simulink model "singletrack_ideal_model_ROS"  (R2018b)
settings: Solver=VariableStepAuto  StartTime=0.0  StopTime=20.0  FixedStep=1e-5  RelTol=1e-3
model workspace (MAT data in the model file):
  SL_ROS_VariableLengthArrays_MaxSizes.CommonInfo.ArrayTruncateAction = 'EmitWarning'
  SL_ROS_VariableLengthArrays_MaxSizes.MsgTypeMap = containers.Map
  SL_ROS_VariableLengthArrays_MaxSizes.MsgTypeMap.serialization.keys = {}
  SL_ROS_VariableLengthArrays_MaxSizes.MsgTypeMap.serialization.values = {}
  SL_ROS_VariableLengthArrays_MaxSizes.MsgTypeMap.serialization.uniformity = 0
  SL_ROS_VariableLengthArrays_MaxSizes.MsgTypeMap.serialization.keyType = 'char'
  SL_ROS_VariableLengthArrays_MaxSizes.MsgTypeMap.serialization.valueType = 'any'
values from neighbouring files (symbols this model uses):
  car_param = [a, b, Cf, Cr, Iz, m]    [init_singletrack.m]
  car_state0 = [psi0, r0, beta0, x0, y0]    [init_singletrack.m]
  fblin_Ts = 0.01    [init_singletrack.m]
  meas_Ts = 0.001    [init_singletrack.m]
  P = 0.5    [init_singletrack.m]    (also in init_unicycle.m)
  ROS_clockPublishingPeriod = 1.0e-2    (= 0.01)    [initParameters.m]    (also in init_singletrack.m = 0.0005)
  ROS_statePublishingPeriod = 2.0e-2    (= 0.02)    [initParameters.m]    (also in init_singletrack.m = 0.01)
undefined symbols (not defined in the file or in its folder): Clock_, fblin_output_singletrack_lopez1, fblin_output_singletrack_lopez2, fblin_output_singletrack_spaliviero, fblin_outputInverse_singletrack_lopez1, fblin_outputInverse_singletrack_lopez2, fblin_outputInverse_singletrack_spaliviero, Sideslip, singleTrack_model, Theta, Vx, Vy, X, Y
libraries: robotlib x14
settings Model: Creator=bascetta  LastModifiedBy=bascetta
settings SFSimCC: SimUseLocalCustomCode=off
settings RTWCC: RTWUseLocalCustomCode=off

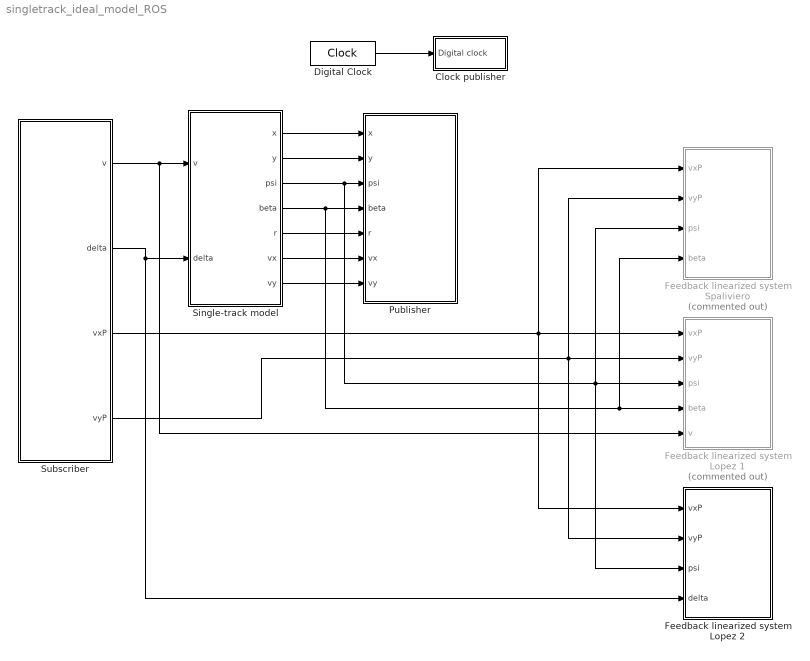
== system singletrack_ideal_model_ROS ==
  Clock publisher : Subsystem
  Digital Clock : DigitalClock  SampleTime=ROS_clockPublishingPeriod
  Feedback linearized system Lopez 1 : Subsystem  Commented=on
  Feedback linearized system Lopez 2 : Subsystem
  Feedback linearized system Spaliviero : Subsystem  Commented=on
  Publisher : Subsystem
  Single-track model : Subsystem  mask{car_parameters=car_param, car_state0=car_state0}
      mask prompts: car_parameters "Car parameters"; car_state0 "Car initial state"
  Subscriber : Subsystem
  wires:
  Single-track model/3(psi) -> Feedback linearized system Lopez 2/3(psi), Feedback linearized system Spaliviero/3(psi), Feedback linearized system Lopez 1/3(psi), Publisher/3(psi)
  Single-track model/4(beta) -> Feedback linearized system Spaliviero/4(beta), Feedback linearized system Lopez 1/4(beta), Publisher/4(beta)
  Subscriber/1(v) -> Feedback linearized system Lopez 1/5(v), Single-track model/1(v)
  Subscriber/2(delta) -> Feedback linearized system Lopez 2/4(delta), Single-track model/2(delta)
  Single-track model/5(r) -> Publisher/5(r)
  Single-track model/2(y) -> Publisher/2(y)
  Single-track model/1(x) -> Publisher/1(x)
  Digital Clock/1 -> Clock publisher/1(Digital clock)
  Subscriber/3(vxP) -> Feedback linearized system Lopez 2/1(vxP), Feedback linearized system Spaliviero/1(vxP), Feedback linearized system Lopez 1/1(vxP)
  Subscriber/4(vyP) -> Feedback linearized system Spaliviero/2(vyP), Feedback linearized system Lopez 2/2(vyP), Feedback linearized system Lopez 1/2(vyP)
  Single-track model/7(vy) -> Publisher/7(vy)
  Single-track model/6(vx) -> Publisher/6(vx)

== system singletrack_ideal_model_ROS/Clock publisher ==
  Digital clock : Inport
  Bus Assignment : BusAssignment  DialogController=Simulink.DDGSource_BusAssignment  AssignedSignals=Clock_.Sec,Clock_.Nsec
  Clock message : robotlib/Blank Message  messageClass=Message  entityType=rosgraph_msgs/Clock  messageType=rosgraph_msgs/Clock  SampleTime=inf
      settings: SourceProductBaseCode=RO
  Clock publishing period : DiscretePulseGenerator  PulseType=Time based  Period=ROS_clockPublishingPeriod  PulseWidth=50
  Publisher : Subsystem  TreatAsAtomicUnit=on
  Time conversion : MATLAB Function  TreatAsAtomicUnit=on
  To Workspace2 : ToWorkspace  VariableName=t  SampleTime=meas_Ts
      settings: Save2DSignal=2-D array (concatenate along first dimension)
  wires:
  Clock message/1 -> Bus Assignment/1
  Bus Assignment/1 -> Publisher/1(clock)
  Time conversion/1(sec) -> Bus Assignment/2
  Time conversion/2(nsec) -> Bus Assignment/3
  Digital clock/1 -> To Workspace2/1, Time conversion/1(digital_time)
  Clock publishing period/1 -> Publisher/Trigger

== system singletrack_ideal_model_ROS/Feedback linearized system Lopez 1 ==
  vxP : Inport
  vyP : Inport  Port=2
  psi : Inport  Port=3
  beta : Inport  Port=4
  v : Inport  Port=5
  Feedback linearized system : Subsystem  mask{car_initial_state=car_state0, P_dist=P, car_parameters=car_param}
      mask prompts: car_initial_state "Car initial state"; P_dist "Point P distance"; car_parameters "Car parameters"
  To Workspace1 : ToWorkspace  VariableName=x_id  SampleTime=meas_Ts
      settings: Save2DSignal=2-D array (concatenate along first dimension)
  To Workspace11 : ToWorkspace  VariableName=xP_id  SampleTime=meas_Ts
      settings: Save2DSignal=2-D array (concatenate along first dimension)
  To Workspace12 : ToWorkspace  VariableName=yP_id  SampleTime=meas_Ts
      settings: Save2DSignal=2-D array (concatenate along first dimension)
  To Workspace2 : ToWorkspace  VariableName=y_id  SampleTime=meas_Ts
      settings: Save2DSignal=2-D array (concatenate along first dimension)
  wires:
  Feedback linearized system/3(x) -> To Workspace1/1
  Feedback linearized system/4(y) -> To Workspace2/1
  vxP/1 -> Feedback linearized system/1(vxp)
  vyP/1 -> Feedback linearized system/2(vyp)
  Feedback linearized system/2(yp) -> To Workspace12/1
  Feedback linearized system/1(xp) -> To Workspace11/1
  psi/1 -> Feedback linearized system/3(psi)
  beta/1 -> Feedback linearized system/4(beta)
  v/1 -> Feedback linearized system/5(v)

== system singletrack_ideal_model_ROS/Feedback linearized system Lopez 2 ==
  vxP : Inport
  vyP : Inport  Port=2
  psi : Inport  Port=3
  delta : Inport  Port=4
  Feedback linearized system : Subsystem  mask{car_initial_state=car_state0, P_dist=P, car_parameters=car_param}
      mask prompts: car_initial_state "Car initial state"; P_dist "Point P distance"; car_parameters "Car parameters"
  To Workspace1 : ToWorkspace  VariableName=x_id  SampleTime=meas_Ts
      settings: Save2DSignal=2-D array (concatenate along first dimension)
  To Workspace11 : ToWorkspace  VariableName=xP_id  SampleTime=meas_Ts
      settings: Save2DSignal=2-D array (concatenate along first dimension)
  To Workspace12 : ToWorkspace  VariableName=yP_id  SampleTime=meas_Ts
      settings: Save2DSignal=2-D array (concatenate along first dimension)
  To Workspace2 : ToWorkspace  VariableName=y_id  SampleTime=meas_Ts
      settings: Save2DSignal=2-D array (concatenate along first dimension)
  wires:
  delta/1 -> Feedback linearized system/4(delta)
  psi/1 -> Feedback linearized system/3(psi)
  Feedback linearized system/1(xp) -> To Workspace11/1
  Feedback linearized system/2(yp) -> To Workspace12/1
  vyP/1 -> Feedback linearized system/2(vyp)
  vxP/1 -> Feedback linearized system/1(vxp)
  Feedback linearized system/4(y) -> To Workspace2/1
  Feedback linearized system/3(x) -> To Workspace1/1

== system singletrack_ideal_model_ROS/Feedback linearized system Spaliviero ==
  vxP : Inport
  vyP : Inport  Port=2
  psi : Inport  Port=3
  beta : Inport  Port=4
  Feedback linearized system : Subsystem  mask{car_initial_state=car_state0, P_dist=P}
      mask prompts: car_initial_state "Car initial state"; P_dist "Point P distance"
  To Workspace1 : ToWorkspace  VariableName=x_id  SampleTime=meas_Ts
      settings: Save2DSignal=2-D array (concatenate along first dimension)
  To Workspace11 : ToWorkspace  VariableName=xP_id  SampleTime=meas_Ts
      settings: Save2DSignal=2-D array (concatenate along first dimension)
  To Workspace12 : ToWorkspace  VariableName=yP_id  SampleTime=meas_Ts
      settings: Save2DSignal=2-D array (concatenate along first dimension)
  To Workspace2 : ToWorkspace  VariableName=y_id  SampleTime=meas_Ts
      settings: Save2DSignal=2-D array (concatenate along first dimension)
  wires:
  Feedback linearized system/1(xp) -> To Workspace11/1
  Feedback linearized system/2(yp) -> To Workspace12/1
  vyP/1 -> Feedback linearized system/2(vyp)
  vxP/1 -> Feedback linearized system/1(vxp)
  Feedback linearized system/4(y) -> To Workspace2/1
  Feedback linearized system/3(x) -> To Workspace1/1
  psi/1 -> Feedback linearized system/3(psi)
  beta/1 -> Feedback linearized system/4(beta)

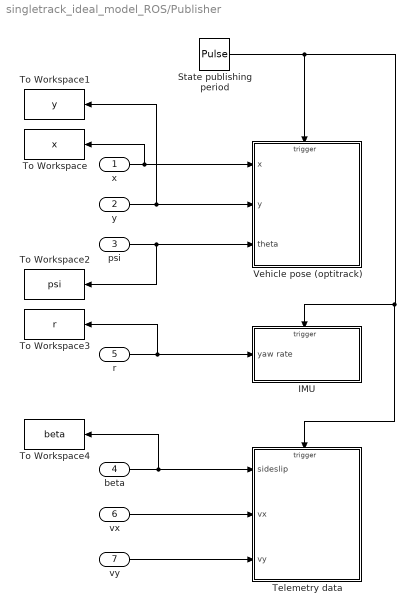
== system singletrack_ideal_model_ROS/Publisher ==
  x : Inport
  y : Inport  Port=2
  psi : Inport  Port=3
  beta : Inport  Port=4
  r : Inport  Port=5
  vx : Inport  Port=6
  vy : Inport  Port=7
  IMU : Subsystem  TreatAsAtomicUnit=on
  State publishing period : DiscretePulseGenerator  PulseType=Time based  Period=ROS_statePublishingPeriod  PulseWidth=50
  Telemetry data : Subsystem  TreatAsAtomicUnit=on
  To Workspace : ToWorkspace  VariableName=x  SampleTime=meas_Ts
      settings: Save2DSignal=2-D array (concatenate along first dimension)
  To Workspace1 : ToWorkspace  VariableName=y  SampleTime=meas_Ts
      settings: Save2DSignal=2-D array (concatenate along first dimension)
  To Workspace2 : ToWorkspace  VariableName=psi  SampleTime=meas_Ts
      settings: Save2DSignal=2-D array (concatenate along first dimension)
  To Workspace3 : ToWorkspace  VariableName=r  SampleTime=meas_Ts
      settings: Save2DSignal=2-D array (concatenate along first dimension)
  To Workspace4 : ToWorkspace  VariableName=beta  SampleTime=meas_Ts
      settings: Save2DSignal=2-D array (concatenate along first dimension)
  Vehicle pose (optitrack) : Subsystem  TreatAsAtomicUnit=on
  wires:
  State publishing period/1 -> Telemetry data/Trigger, IMU/Trigger, Vehicle pose (optitrack)/Trigger
  x/1 -> To Workspace/1, Vehicle pose (optitrack)/1(x)
  y/1 -> To Workspace1/1, Vehicle pose (optitrack)/2(y)
  psi/1 -> To Workspace2/1, Vehicle pose (optitrack)/3(theta)
  r/1 -> To Workspace3/1, IMU/1(yaw rate)
  beta/1 -> Telemetry data/1(sideslip), To Workspace4/1
  vy/1 -> Telemetry data/3(vy)
  vx/1 -> Telemetry data/2(vx)

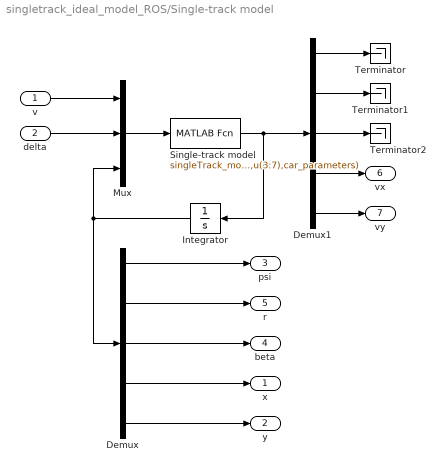
== system singletrack_ideal_model_ROS/Single-track model ==
  v : Inport
  delta : Inport  Port=2
  Demux : Demux  Outputs=5
  Demux1 : Demux  Outputs=5
  Integrator : Integrator  InitialCondition=car_state0
  Mux : Mux  Inputs=3
  Single-track model : MATLABFcn  MATLABFcn=singleTrack_model(u(1:2),u(3:7),car_parameters)  OutputDimensions=5
  Terminator : Terminator
  Terminator1 : Terminator
  Terminator2 : Terminator
  x : Outport
  y : Outport  Port=2
  psi : Outport  Port=3
  beta : Outport  Port=4
  r : Outport  Port=5
  vx : Outport  Port=6
  vy : Outport  Port=7
  wires:
  Integrator/1 -> Demux/1, Mux/3
  Single-track model/1 -> Demux1/1, Integrator/1
  Mux/1 -> Single-track model/1
  Demux/3 -> beta/1
  v/1 -> Mux/1
  delta/1 -> Mux/2
  Demux/5 -> y/1
  Demux/4 -> x/1
  Demux/2 -> r/1
  Demux/1 -> psi/1
  Demux1/2 -> Terminator1/1
  Demux1/1 -> Terminator/1
  Demux1/3 -> Terminator2/1
  Demux1/4 -> vx/1
  Demux1/5 -> vy/1

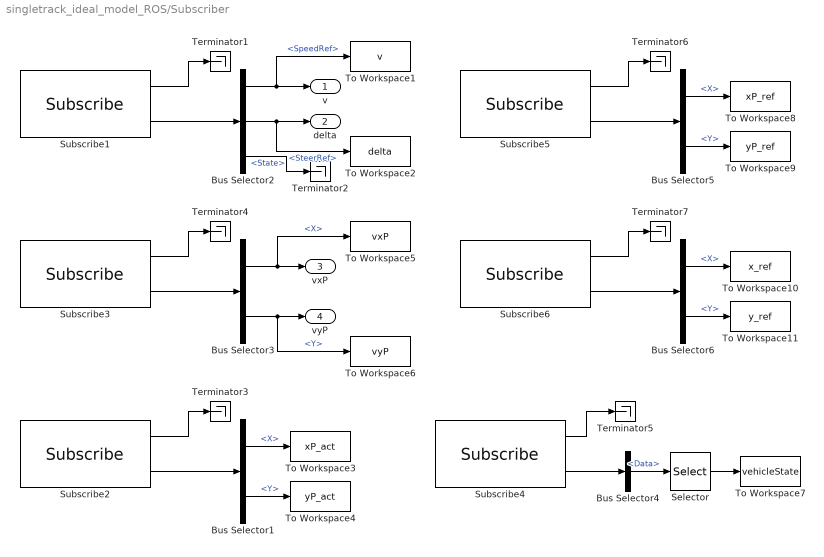
== system singletrack_ideal_model_ROS/Subscriber ==
  Bus Selector1 : BusSelector  OutputSignals=Point.X,Point.Y
  Bus Selector2 : BusSelector  OutputSignals=SpeedRef,SteerRef,State
  Bus Selector3 : BusSelector  OutputSignals=Twist.Linear.X,Twist.Linear.Y
  Bus Selector4 : BusSelector  OutputSignals=Data
  Bus Selector5 : BusSelector  OutputSignals=Point.X,Point.Y
  Bus Selector6 : BusSelector  OutputSignals=Point.X,Point.Y
  Selector : Selector  InputPortWidth=128  IndexOptions=Starting index (dialog)  Indices=1  OutputSizes=9
  Subscribe1 : robotlib/Subscribe  topicSource=Specify your own  topic=/controller_cmd  messageType=car_msgs/car_cmd  sampleTime=-1  messageQueueLength=1
      settings: SourceProductBaseCode=RO
  Subscribe2 : robotlib/Subscribe  topicSource=Specify your own  topic=/feedback_linearization/pointP_actPos  messageType=geometry_msgs/PointStamped  sampleTime=-1  messageQueueLength=1
      settings: SourceProductBaseCode=RO
  Subscribe3 : robotlib/Subscribe  topicSource=Specify your own  topic=/feedback_linearization/pointP_actVel  messageType=geometry_msgs/TwistStamped  sampleTime=-1  messageQueueLength=1
      settings: SourceProductBaseCode=RO
  Subscribe4 : robotlib/Subscribe  topicSource=Specify your own  topic=/feedback_linearization/vehicleState  messageType=std_msgs/Float64MultiArray  sampleTime=-1  messageQueueLength=1
      settings: SourceProductBaseCode=RO
  Subscribe5 : robotlib/Subscribe  topicSource=Specify your own  topic=/feedback_linearization/pointP_refPos  messageType=geometry_msgs/PointStamped  sampleTime=-1  messageQueueLength=1
      settings: SourceProductBaseCode=RO
  Subscribe6 : robotlib/Subscribe  topicSource=Specify your own  topic=/feedback_linearization/vehicle_refPos  messageType=geometry_msgs/PointStamped  sampleTime=-1  messageQueueLength=1
      settings: SourceProductBaseCode=RO
  Terminator{1..7} (7 alike) : Terminator
  To Workspace1 : ToWorkspace  VariableName=v  SampleTime=meas_Ts
      settings: Save2DSignal=2-D array (concatenate along first dimension)
  To Workspace10 : ToWorkspace  VariableName=x_ref  SampleTime=meas_Ts
      settings: Save2DSignal=2-D array (concatenate along first dimension)
  To Workspace11 : ToWorkspace  VariableName=y_ref  SampleTime=meas_Ts
      settings: Save2DSignal=2-D array (concatenate along first dimension)
  To Workspace2 : ToWorkspace  VariableName=delta  SampleTime=meas_Ts
      settings: Save2DSignal=2-D array (concatenate along first dimension)
  To Workspace3 : ToWorkspace  VariableName=xP_act  SampleTime=meas_Ts
      settings: Save2DSignal=2-D array (concatenate along first dimension)
  To Workspace4 : ToWorkspace  VariableName=yP_act  SampleTime=meas_Ts
      settings: Save2DSignal=2-D array (concatenate along first dimension)
  To Workspace5 : ToWorkspace  VariableName=vxP  SampleTime=meas_Ts
      settings: Save2DSignal=2-D array (concatenate along first dimension)
  To Workspace6 : ToWorkspace  VariableName=vyP  SampleTime=meas_Ts
      settings: Save2DSignal=2-D array (concatenate along first dimension)
  To Workspace7 : ToWorkspace  VariableName=vehicleState  SampleTime=meas_Ts
      settings: Save2DSignal=2-D array (concatenate along first dimension)
  To Workspace8 : ToWorkspace  VariableName=xP_ref  SampleTime=meas_Ts
      settings: Save2DSignal=2-D array (concatenate along first dimension)
  To Workspace9 : ToWorkspace  VariableName=yP_ref  SampleTime=meas_Ts
      settings: Save2DSignal=2-D array (concatenate along first dimension)
  v : Outport
  delta : Outport  Port=2
  vxP : Outport  Port=3
  vyP : Outport  Port=4
  wires:
  Subscribe1/1 -> Terminator1/1
  Subscribe1/2 -> Bus Selector2/1
  Bus Selector2/1 -> To Workspace1/1, v/1  "<SpeedRef>"
  Bus Selector2/2 -> To Workspace2/1, delta/1  "<SteerRef>"
  Bus Selector2/3 -> Terminator2/1  "<State>"
  Subscribe2/1 -> Terminator3/1
  Subscribe2/2 -> Bus Selector1/1
  Bus Selector1/1 -> To Workspace3/1  "<X>"
  Bus Selector1/2 -> To Workspace4/1  "<Y>"
  Bus Selector3/2 -> vyP/1, To Workspace6/1  "<Y>"
  Subscribe3/1 -> Terminator4/1
  Bus Selector3/1 -> vxP/1, To Workspace5/1  "<X>"
  Subscribe4/1 -> Terminator5/1
  Subscribe4/2 -> Bus Selector4/1
  Bus Selector4/1 -> Selector/1  "<Data>"
  Selector/1 -> To Workspace7/1
  Subscribe5/1 -> Terminator6/1
  Bus Selector5/1 -> To Workspace8/1  "<X>"
  Bus Selector5/2 -> To Workspace9/1  "<Y>"
  Subscribe5/2 -> Bus Selector5/1
  Subscribe3/2 -> Bus Selector3/1
  Subscribe6/1 -> Terminator7/1
  Bus Selector6/1 -> To Workspace10/1  "<X>"
  Bus Selector6/2 -> To Workspace11/1  "<Y>"
  Subscribe6/2 -> Bus Selector6/1

== system singletrack_ideal_model_ROS/Clock publisher/Publisher ==
  clock : Inport
  Trigger : TriggerPort  VariantControl=Variant
  Publish : robotlib/Publish  topicSource=Specify your own  topic=/clock  messageType=rosgraph_msgs/Clock  messageQueueLength=1
      settings: SourceProductBaseCode=RO
  wires:
  clock/1 -> Publish/1

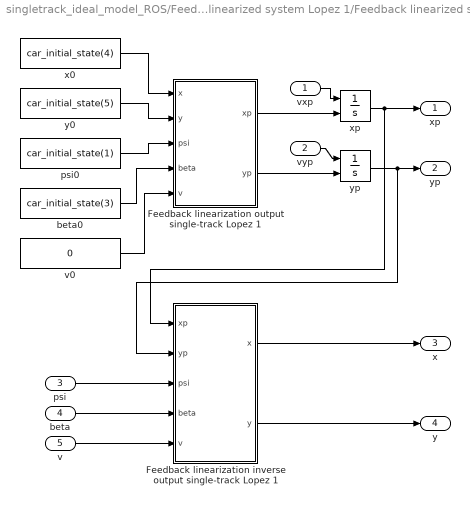
== system singletrack_ideal_model_ROS/Feedback linearized system Lopez 1/Feedback linearized system ==
  vxp : Inport
  vyp : Inport  Port=2
  psi : Inport  Port=3
  beta : Inport  Port=4
  v : Inport  Port=5
  " xp " : Integrator  InitialConditionSource=external  InitialCondition=car_state0(4)
  " yp " : Integrator  InitialConditionSource=external  InitialCondition=car_state0(5)
  Feedback linearization inverse output single-track Lopez 1 : Subsystem  mask{P_dist=P_dist, car_parameters=car_parameters}
      mask prompts: P_dist "Distance of point P"; car_parameters "Car parameters"
  Feedback linearization output single-track Lopez 1 : Subsystem  mask{P_dist=P_dist, car_parameters=car_parameters}
      mask prompts: P_dist "Distance of point P"; car_parameters "Car parameters"
  beta0 : Constant  Value=car_initial_state(3)
  psi0 : Constant  Value=car_initial_state(1)
  v0 : Constant  Value=0
  x0 : Constant  Value=car_initial_state(4)
  y0 : Constant  Value=car_initial_state(5)
  xp : Outport
  yp : Outport  Port=2
  x : Outport  Port=3
  y : Outport  Port=4
  wires:
  Feedback linearization inverse output single-track Lopez 1/1(x) -> x/1
  Feedback linearization inverse output single-track Lopez 1/2(y) -> y/1
  beta0/1 -> Feedback linearization output single-track Lopez 1/4(beta)
  psi0/1 -> Feedback linearization output single-track Lopez 1/3(psi)
  y0/1 -> Feedback linearization output single-track Lopez 1/2(y)
  x0/1 -> Feedback linearization output single-track Lopez 1/1(x)
  Feedback linearization output single-track Lopez 1/2(yp) -> " yp "/2
  Feedback linearization output single-track Lopez 1/1(xp) -> " xp "/2
  " xp "/1 -> xp/1, Feedback linearization inverse output single-track Lopez 1/1(xp)
  " yp "/1 -> yp/1, Feedback linearization inverse output single-track Lopez 1/2(yp)
  vxp/1 -> " xp "/1
  vyp/1 -> " yp "/1
  psi/1 -> Feedback linearization inverse output single-track Lopez 1/3(psi)
  beta/1 -> Feedback linearization inverse output single-track Lopez 1/4(beta)
  v0/1 -> Feedback linearization output single-track Lopez 1/5(v)
  v/1 -> Feedback linearization inverse output single-track Lopez 1/5(v)

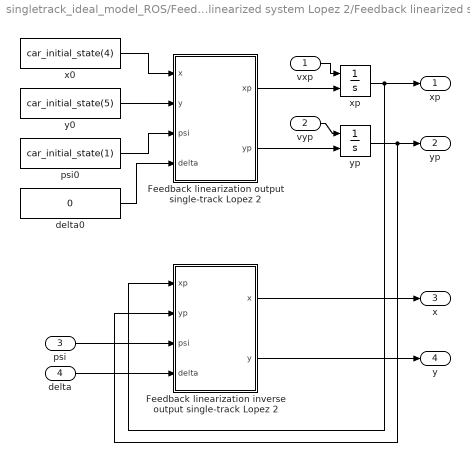
== system singletrack_ideal_model_ROS/Feedback linearized system Lopez 2/Feedback linearized system ==
  vxp : Inport
  vyp : Inport  Port=2
  psi : Inport  Port=3
  delta : Inport  Port=4
  " xp " : Integrator  InitialConditionSource=external  InitialCondition=car_state0(4)
  " yp " : Integrator  InitialConditionSource=external  InitialCondition=car_state0(5)
  Feedback linearization inverse output single-track Lopez 2 : Subsystem  mask{P_dist=P_dist, car_parameters=car_parameters}
      mask prompts: P_dist "Distance of point P"; car_parameters "Car parameters"
  Feedback linearization output single-track Lopez 2 : Subsystem  mask{P_dist=P_dist, car_parameters=car_parameters}
      mask prompts: P_dist "Distance of point P"; car_parameters "Car parameters"
  delta0 : Constant  Value=0
  psi0 : Constant  Value=car_initial_state(1)
  x0 : Constant  Value=car_initial_state(4)
  y0 : Constant  Value=car_initial_state(5)
  xp : Outport
  yp : Outport  Port=2
  x : Outport  Port=3
  y : Outport  Port=4
  wires:
  delta/1 -> Feedback linearization inverse output single-track Lopez 2/4(delta)
  psi/1 -> Feedback linearization inverse output single-track Lopez 2/3(psi)
  vyp/1 -> " yp "/1
  vxp/1 -> " xp "/1
  " yp "/1 -> Feedback linearization inverse output single-track Lopez 2/2(yp), yp/1
  " xp "/1 -> Feedback linearization inverse output single-track Lopez 2/1(xp), xp/1
  Feedback linearization output single-track Lopez 2/1(xp) -> " xp "/2
  Feedback linearization output single-track Lopez 2/2(yp) -> " yp "/2
  x0/1 -> Feedback linearization output single-track Lopez 2/1(x)
  y0/1 -> Feedback linearization output single-track Lopez 2/2(y)
  psi0/1 -> Feedback linearization output single-track Lopez 2/3(psi)
  delta0/1 -> Feedback linearization output single-track Lopez 2/4(delta)
  Feedback linearization inverse output single-track Lopez 2/2(y) -> y/1
  Feedback linearization inverse output single-track Lopez 2/1(x) -> x/1

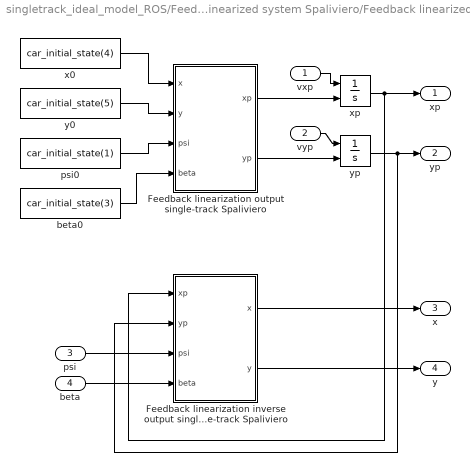
== system singletrack_ideal_model_ROS/Feedback linearized system Spaliviero/Feedback linearized system ==
  vxp : Inport
  vyp : Inport  Port=2
  psi : Inport  Port=3
  beta : Inport  Port=4
  " xp " : Integrator  InitialConditionSource=external  InitialCondition=car_state0(4)
  " yp " : Integrator  InitialConditionSource=external  InitialCondition=car_state0(5)
  Feedback linearization inverse output single-track Spaliviero : Subsystem  mask{P_dist=P_dist}
      mask prompts: P_dist "Distance of point P"
  Feedback linearization output single-track Spaliviero : Subsystem  mask{P_dist=P_dist}
      mask prompts: P_dist "Distance of point P"
  beta0 : Constant  Value=car_initial_state(3)
  psi0 : Constant  Value=car_initial_state(1)
  x0 : Constant  Value=car_initial_state(4)
  y0 : Constant  Value=car_initial_state(5)
  xp : Outport
  yp : Outport  Port=2
  x : Outport  Port=3
  y : Outport  Port=4
  wires:
  vyp/1 -> " yp "/1
  vxp/1 -> " xp "/1
  " yp "/1 -> Feedback linearization inverse output single-track Spaliviero/2(yp), yp/1
  " xp "/1 -> Feedback linearization inverse output single-track Spaliviero/1(xp), xp/1
  Feedback linearization output single-track Spaliviero/1(xp) -> " xp "/2
  Feedback linearization output single-track Spaliviero/2(yp) -> " yp "/2
  x0/1 -> Feedback linearization output single-track Spaliviero/1(x)
  y0/1 -> Feedback linearization output single-track Spaliviero/2(y)
  psi0/1 -> Feedback linearization output single-track Spaliviero/3(psi)
  beta0/1 -> Feedback linearization output single-track Spaliviero/4(beta)
  Feedback linearization inverse output single-track Spaliviero/2(y) -> y/1
  Feedback linearization inverse output single-track Spaliviero/1(x) -> x/1
  psi/1 -> Feedback linearization inverse output single-track Spaliviero/3(psi)
  beta/1 -> Feedback linearization inverse output single-track Spaliviero/4(beta)

== system singletrack_ideal_model_ROS/Publisher/IMU ==
  yaw rate : Inport
  Trigger : TriggerPort  VariantControl=Variant
  Blank Message : robotlib/Blank Message  messageClass=Message  entityType=sensor_msgs/Imu  messageType=sensor_msgs/Imu  SampleTime=inf
      settings: SourceProductBaseCode=RO
  Bus Assignment : BusAssignment  DialogController=Simulink.DDGSource_BusAssignment  AssignedSignals=AngularVelocity.Z
  Publish : robotlib/Publish  topicSource=Specify your own  topic=/imu/data  messageType=sensor_msgs/Imu  messageQueueLength=1
      settings: SourceProductBaseCode=RO
  wires:
  Blank Message/1 -> Bus Assignment/1
  Bus Assignment/1 -> Publish/1
  yaw rate/1 -> Bus Assignment/2

== system singletrack_ideal_model_ROS/Publisher/Telemetry data ==
  sideslip : Inport
  vx : Inport  Port=2
  vy : Inport  Port=3
  Trigger : TriggerPort  VariantControl=Variant
  Blank Message : robotlib/Blank Message  messageClass=Message  entityType=car_msgs/simulated_telemetry  messageType=car_msgs/simulated_telemetry  SampleTime=inf
      settings: SourceProductBaseCode=RO
  Bus Assignment : BusAssignment  DialogController=Simulink.DDGSource_BusAssignment  AssignedSignals=Sideslip,Vx,Vy
  Publish : robotlib/Publish  topicSource=Specify your own  topic=/car_simulator/telemetry  messageType=car_msgs/simulated_telemetry  messageQueueLength=1
      settings: SourceProductBaseCode=RO
  wires:
  Bus Assignment/1 -> Publish/1
  Blank Message/1 -> Bus Assignment/1
  sideslip/1 -> Bus Assignment/2
  vx/1 -> Bus Assignment/3
  vy/1 -> Bus Assignment/4

== system singletrack_ideal_model_ROS/Publisher/Vehicle pose (optitrack) ==
  x : Inport
  y : Inport  Port=2
  theta : Inport  Port=3
  Trigger : TriggerPort  VariantControl=Variant
  Blank Message : robotlib/Blank Message  messageClass=Message  entityType=geometry_msgs/Pose2D  messageType=geometry_msgs/Pose2D  SampleTime=inf
      settings: SourceProductBaseCode=RO
  Bus Assignment : BusAssignment  DialogController=Simulink.DDGSource_BusAssignment  AssignedSignals=X,Y,Theta
  Publish : robotlib/Publish  topicSource=Specify your own  topic=/car/ground_pose  messageType=geometry_msgs/Pose2D  messageQueueLength=1
      settings: SourceProductBaseCode=RO
  wires:
  Blank Message/1 -> Bus Assignment/1
  Bus Assignment/1 -> Publish/1
  x/1 -> Bus Assignment/2
  y/1 -> Bus Assignment/3
  theta/1 -> Bus Assignment/4

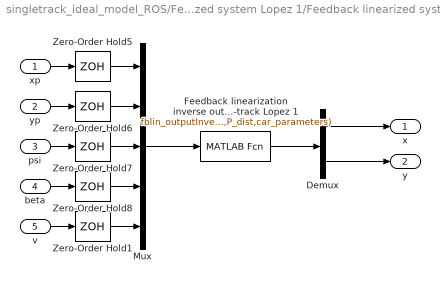
== system singletrack_ideal_model_ROS/Feedback linearized system Lopez 1/Feedback linearized system/Feedback linearization inverse output single-track Lopez 1 ==
  xp : Inport
  yp : Inport  Port=2
  psi : Inport  Port=3
  beta : Inport  Port=4
  v : Inport  Port=5
  Demux : Demux  Outputs=2
  Feedback linearization inverse output single-track Lopez 1 : MATLABFcn  MATLABFcn=fblin_outputInverse_singletrack_lopez1(u(1),u(2),u(3),u(4),u(5),P_dist,car_parameters)  OutputDimensions=2
  Mux : Mux  Inputs=5
  Zero-Order Hold{1,5..8} (5 alike) : ZeroOrderHold  SampleTime=fblin_Ts
  x : Outport
  y : Outport  Port=2
  wires:
  yp/1 -> Zero-Order Hold6/1
  Demux/2 -> y/1
  Feedback linearization inverse output single-track Lopez 1/1 -> Demux/1
  Demux/1 -> x/1
  Mux/1 -> Feedback linearization inverse output single-track Lopez 1/1
  xp/1 -> Zero-Order Hold5/1
  Zero-Order Hold5/1 -> Mux/1
  Zero-Order Hold8/1 -> Mux/4
  Zero-Order Hold7/1 -> Mux/3
  Zero-Order Hold6/1 -> Mux/2
  psi/1 -> Zero-Order Hold7/1
  beta/1 -> Zero-Order Hold8/1
  v/1 -> Zero-Order Hold1/1
  Zero-Order Hold1/1 -> Mux/5

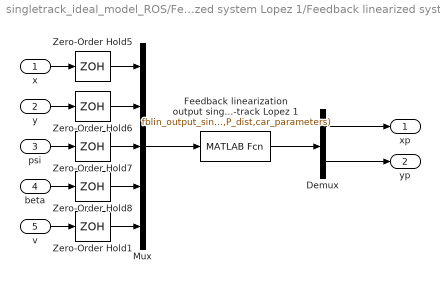
== system singletrack_ideal_model_ROS/Feedback linearized system Lopez 1/Feedback linearized system/Feedback linearization output single-track Lopez 1 ==
  x : Inport
  y : Inport  Port=2
  psi : Inport  Port=3
  beta : Inport  Port=4
  v : Inport  Port=5
  Demux : Demux  Outputs=2
  Feedback linearization output single-track Lopez 1 : MATLABFcn  MATLABFcn=fblin_output_singletrack_lopez1(u(1),u(2),u(3),u(4),u(5),P_dist,car_parameters)  OutputDimensions=2
  Mux : Mux  Inputs=5
  Zero-Order Hold{1,5..8} (5 alike) : ZeroOrderHold  SampleTime=fblin_Ts
  xp : Outport
  yp : Outport  Port=2
  wires:
  Zero-Order Hold6/1 -> Mux/2
  Zero-Order Hold7/1 -> Mux/3
  Zero-Order Hold8/1 -> Mux/4
  Zero-Order Hold5/1 -> Mux/1
  x/1 -> Zero-Order Hold5/1
  Mux/1 -> Feedback linearization output single-track Lopez 1/1
  Demux/1 -> xp/1
  Feedback linearization output single-track Lopez 1/1 -> Demux/1
  Demux/2 -> yp/1
  y/1 -> Zero-Order Hold6/1
  v/1 -> Zero-Order Hold1/1
  Zero-Order Hold1/1 -> Mux/5
  beta/1 -> Zero-Order Hold8/1
  psi/1 -> Zero-Order Hold7/1

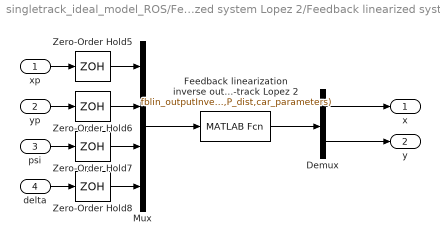
== system singletrack_ideal_model_ROS/Feedback linearized system Lopez 2/Feedback linearized system/Feedback linearization inverse output single-track Lopez 2 ==
  xp : Inport
  yp : Inport  Port=2
  psi : Inport  Port=3
  delta : Inport  Port=4
  Demux : Demux  Outputs=2
  Feedback linearization inverse output single-track Lopez 2 : MATLABFcn  MATLABFcn=fblin_outputInverse_singletrack_lopez2(u(1),u(2),u(3),u(4),P_dist,car_parameters)  OutputDimensions=2
  Mux : Mux
  Zero-Order Hold{5..8} (4 alike) : ZeroOrderHold  SampleTime=fblin_Ts
  x : Outport
  y : Outport  Port=2
  wires:
  delta/1 -> Zero-Order Hold8/1
  psi/1 -> Zero-Order Hold7/1
  Zero-Order Hold6/1 -> Mux/2
  Zero-Order Hold7/1 -> Mux/3
  Zero-Order Hold8/1 -> Mux/4
  Zero-Order Hold5/1 -> Mux/1
  xp/1 -> Zero-Order Hold5/1
  Mux/1 -> Feedback linearization inverse output single-track Lopez 2/1
  Demux/1 -> x/1
  Feedback linearization inverse output single-track Lopez 2/1 -> Demux/1
  Demux/2 -> y/1
  yp/1 -> Zero-Order Hold6/1

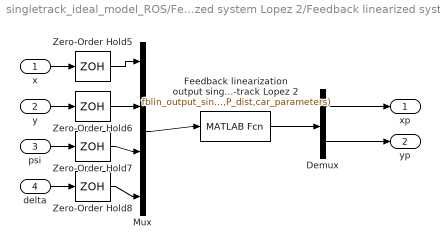
== system singletrack_ideal_model_ROS/Feedback linearized system Lopez 2/Feedback linearized system/Feedback linearization output single-track Lopez 2 ==
  x : Inport
  y : Inport  Port=2
  psi : Inport  Port=3
  delta : Inport  Port=4
  Demux : Demux  Outputs=2
  Feedback linearization output single-track Lopez 2 : MATLABFcn  MATLABFcn=fblin_output_singletrack_lopez2(u(1),u(2),u(3),u(4),P_dist,car_parameters)  OutputDimensions=2
  Mux : Mux
  Zero-Order Hold{5..8} (4 alike) : ZeroOrderHold  SampleTime=fblin_Ts
  xp : Outport
  yp : Outport  Port=2
  wires:
  psi/1 -> Zero-Order Hold7/1
  delta/1 -> Zero-Order Hold8/1
  y/1 -> Zero-Order Hold6/1
  Demux/2 -> yp/1
  Feedback linearization output single-track Lopez 2/1 -> Demux/1
  Demux/1 -> xp/1
  Mux/1 -> Feedback linearization output single-track Lopez 2/1
  x/1 -> Zero-Order Hold5/1
  Zero-Order Hold5/1 -> Mux/1
  Zero-Order Hold8/1 -> Mux/4
  Zero-Order Hold7/1 -> Mux/3
  Zero-Order Hold6/1 -> Mux/2

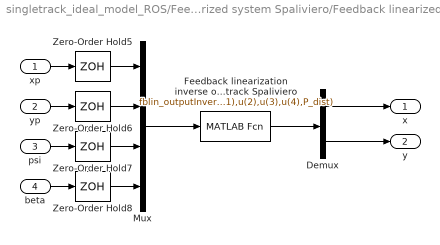
== system singletrack_ideal_model_ROS/Feedback linearized system Spaliviero/Feedback linearized system/Feedback linearization inverse output single-track Spaliviero ==
  xp : Inport
  yp : Inport  Port=2
  psi : Inport  Port=3
  beta : Inport  Port=4
  Demux : Demux  Outputs=2
  Feedback linearization inverse output single-track Spaliviero : MATLABFcn  MATLABFcn=fblin_outputInverse_singletrack_spaliviero(u(1),u(2),u(3),u(4),P_dist)  OutputDimensions=2
  Mux : Mux
  Zero-Order Hold{5..8} (4 alike) : ZeroOrderHold  SampleTime=fblin_Ts
  x : Outport
  y : Outport  Port=2
  wires:
  Zero-Order Hold6/1 -> Mux/2
  Zero-Order Hold7/1 -> Mux/3
  Zero-Order Hold8/1 -> Mux/4
  Zero-Order Hold5/1 -> Mux/1
  xp/1 -> Zero-Order Hold5/1
  Mux/1 -> Feedback linearization inverse output single-track Spaliviero/1
  Demux/1 -> x/1
  Feedback linearization inverse output single-track Spaliviero/1 -> Demux/1
  Demux/2 -> y/1
  yp/1 -> Zero-Order Hold6/1
  psi/1 -> Zero-Order Hold7/1
  beta/1 -> Zero-Order Hold8/1

== system singletrack_ideal_model_ROS/Feedback linearized system Spaliviero/Feedback linearized system/Feedback linearization output single-track Spaliviero ==
  x : Inport
  y : Inport  Port=2
  psi : Inport  Port=3
  beta : Inport  Port=4
  Demux : Demux  Outputs=2
  Feedback linearization output single-track Spaliviero : MATLABFcn  MATLABFcn=fblin_output_singletrack_spaliviero(u(1),u(2),u(3),u(4),P_dist)  OutputDimensions=2
  Mux : Mux
  Zero-Order Hold{5..8} (4 alike) : ZeroOrderHold  SampleTime=fblin_Ts
  xp : Outport
  yp : Outport  Port=2
  wires:
  y/1 -> Zero-Order Hold6/1
  Demux/2 -> yp/1
  Feedback linearization output single-track Spaliviero/1 -> Demux/1
  Demux/1 -> xp/1
  Mux/1 -> Feedback linearization output single-track Spaliviero/1
  x/1 -> Zero-Order Hold5/1
  Zero-Order Hold5/1 -> Mux/1
  Zero-Order Hold8/1 -> Mux/4
  Zero-Order Hold7/1 -> Mux/3
  Zero-Order Hold6/1 -> Mux/2
  psi/1 -> Zero-Order Hold7/1
  beta/1 -> Zero-Order Hold8/1

== matlab function singletrack_ideal_model_ROS/Clock publisher/Time conversion ==
  data: digital_time input; sec output; nsec output
function [sec,nsec] = time2rosclock(digital_time)

sec = floor(digital_time);
nsec = round((digital_time-sec)*1.0e+9);
